simulink model "Sfunction_test"  (Simulink 8.5)
settings: Solver=ode45  StartTime=0.0  StopTime=7  RelTol=1e-3
undefined symbols (not defined in the file or in its folder): sample_time
settings Model: Creator=User  LastModifiedBy=User
settings DataIOCC: SignalLoggingSaveFormat=Dataset
settings OptimizationCC: ExpressionDepthLimit=128
settings DebuggingCC: UnderspecifiedInitializationDetection=Simplified  MergeDetectMultiDrivingBlocksExec=error  FcnCallInpInsideContextMsg=EnableAllAsError  StateNameClashWarn=none
settings GRTTargetCC: CombineOutputUpdateFcns=on  GRTInterface=off

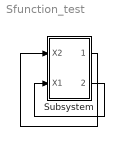
== system Sfunction_test ==
  Subsystem : Subsystem
  wires:
  Subsystem/2(x_1) -> Subsystem/2(X1)
  Subsystem/1(x_22) -> Subsystem/1(X2)

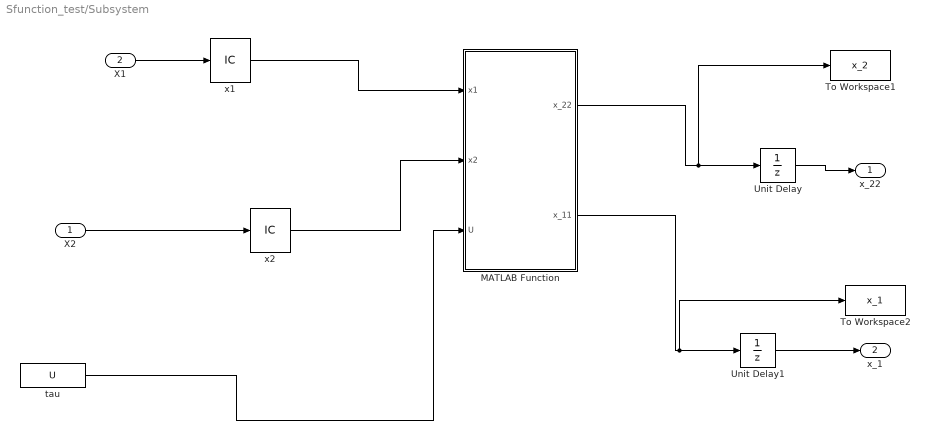
== system Sfunction_test/Subsystem ==
  X2 : Inport  PortDimensions=[7]
  X1 : Inport  Port=2  PortDimensions=[7]
  MATLAB Function : MATLAB Function  TreatAsAtomicUnit=on
  To Workspace1 : ToWorkspace  VariableName=x_2  SaveFormat=Structure With Time  SampleTime=-1
  To Workspace2 : ToWorkspace  VariableName=x_1  SaveFormat=Structure With Time  SampleTime=-1
  Unit Delay : UnitDelay  SampleTime=sample_time
  Unit Delay1 : UnitDelay  SampleTime=sample_time
  "tau " : FromWorkspace  VariableName=U  SampleTime=sample_time
  x1 : InitialCondition  Value=[-0.1106,-1.9490,-0.192,3.18400,0.2825,0.0969,-0.2798]
  x2 : InitialCondition  Value=[0 0 0 0 0 0 0]
  x_22 : Outport  PortDimensions=7
  x_1 : Outport  Port=2  PortDimensions=7
  wires:
  MATLAB Function/1(x_22) -> To Workspace1/1, Unit Delay/1
  MATLAB Function/2(x_11) -> To Workspace2/1, Unit Delay1/1
  "tau "/1 -> MATLAB Function/3(U)
  x1/1 -> MATLAB Function/1(x1)
  x2/1 -> MATLAB Function/2(x2)
  X2/1 -> x2/1
  X1/1 -> x1/1
  Unit Delay/1 -> x_22/1
  Unit Delay1/1 -> x_1/1

== matlab function Subsystem/MATLAB Function ==
  data: x1 input double; x_22 output double; x2 input double; U input double; x_11 output double
%
% gravComp7DOFNum Compute inverse dynamics via recursive Newton-Euler formulation
%
% Recursive Newton-Euler for standard Denavit-Hartenberg notation.
%

% Copyright (C) 1993-2011, by Peter I. Corke
%
% This file originally was part of The Robotics Toolbox for Matlab (RTB).
%
% http://www.petercorke.com

%
% Simplified from rne_dh for 7DOF WAM to compute only torque from gravity by Hans Vorsteveld
% Does not use structures from RTB, only the RNE algorithm
%

function [x_22,x_11] = PID(x1,x2,U)

%-------------------------------------------------------------------------------------
%   SETUP THE ARM
%-------------------------------------------------------------------------------------    
  Ts=0.002;
    



 
 
yd = [posd;veld];


        
         
         
        % In experimental work you do not add noise instead you only use measurement of position
        x_11 =  x2*Ts + x1; % Here we are estimating position using the extimate of x2 and measurement of x1 at present time
        
        %XX2 = (x_11-x_1)/Ts; 
        %XX2 = (x1-x1d)/Ts; 
        
        %x_22= (-inv(D(pos_meas))*((G(pos_meas)))+ inv(D(pos_meas))*U)*Ts + XX2 ;
        x3=(-inv(D(x1))*((G(x1)))+ inv(D(x1))*U);
       x_22=  x2 + Ts*x3;
        
        
        
    
   
end 

function G=G(q)


DH_a = [0 0 0.045 -0.045 0 0 0];
    DH_d = [0 0 .55 0 0.45 0 0.061];
    DH_alpha = [-pi/2 pi/2 -pi/2 pi/2 -pi/2 pi/2 0];

    m = [10.7676 3.87 1.8022 2.4 0.1237 0.4979886 0.07548270];
    
     
    com= zeros(3,7);
    
   com(:,1) = [-0.00443422;0.12189039;-0.00066489];
    com(:,2) = [-0.00236983;0.03105614;0.01542114 ];
    com(:,3) = [-0.03825858;0.20750770;0.00003309];
    com(:,4) = [0.00498512;-0.00022942;0.13271662 ];
    com(:,5) = [0.00008921;0.00511217;0.00435824];
    com(:,6) = [-0.00012262;-0.01703194;0.02468336];
    com(:,7) = [-0.00007974;0.00016313;-0.00323552 ];
     
     % hand_mass =1.385;
      %  DH_d(7) =DH_d(7)+ .0953; % Adding the distance to the hand frame for the Schunk Gripper
       % com(:,7) =(com(:,7).*hand_mass+com(:,7).*m(7))/(hand_mass+m(7)); % Finding the combined center of mass
        %m(7) =m(7)+hand_mass;  
        
    I=zeros(3,3,7);
    T=zeros(4,4,7);
     I(:,:,1) = [0.29486350,-0.00795023,-0.00009311;
                 -0.00795023,0.11350017,-0.00018711;
                -0.00009311,-0.00018711,0.25065343];
    I(:,:,2) =[0.02606840,-0.00001346,-0.00011701;
               -0.00001346,0.01472202,0.00003659;
              -0.00011701,0.00003659,0.01934814];
    I(:,:,3) = [0.13671601,-0.01680434, 0.00000510;
               -0.01680434,0.00588354,-0.00000530;
                0.00000510,-0.00000530,0.13951371];
    I(:,:,4) = [ 0.05719268,0.00001467,0.00008193;
                 0.00001467,0.05716470,-0.00009417;
                 0.00008193,-0.00009417,0.00300441] ;
    I(:,:,5) =[0.00005587,0.00000026,.00000000;
               0.00000026,0.00007817,-0.00000083;
               0.00000000,-0.00000083,0.00006594];
    I(:,:,6) = [0.00093106,0.00000148,-0.00000201;
                0.00000148, 0.00049833,-0.00022162;
               -0.00000201,-0.00022162,0.00057483];
    I(:,:,7) = [0.003167342, 0,0;       % Approximate Inertia Tensor for Schunk Gripper
                0,0.001128942,0;
                 0,0,0.00258007;];  
            
             
for j=1:7,
        a = DH_a(j);
        d = DH_d(j);
        alpha = DH_alpha(j);
        T(:,:,j) = getTransformDH(a, d, alpha, q(j));
end 


comstar=zeros(4,7);

   
    comstar(:,1) = [com(:,1);1];
    comstar(:,2) = [com(:,2);1];
    comstar(:,3) = [com(:,3);1];
    comstar(:,4) = [com(:,4);1];
    comstar(:,5) = [com(:,5);1];
    comstar(:,6) = [com(:,6);1];
    comstar(:,7) = [com(:,7);1];
    
    Q=zeros(4,4);
    
    Q=[0,-1,0,0;
     1,0,0,0;
     0,0,0,0;
     0,0,0,0];
   
 gravity=[0,0,-9.81,0];
 G=zeros(7,1)
 
   G(1)= -m(1)*gravity*Q*T(:,:,1)*comstar(:,1)-m(2)*gravity*Q*T(:,:,1)*T(:,:,2)*comstar(:,2)-m(3)*gravity*Q*T(:,:,1)*T(:,:,2)*T(:,:,3)*comstar(:,3)-m(4)*gravity*Q*T(:,:,1)*T(:,:,2)*T(:,:,3)*T(:,:,4)*comstar(:,4)-m(5)*gravity*Q*T(:,:,1)*T(:,:,2)*T(:,:,3)*T(:,:,4)*T(:,:,5)*comstar(:,5)-m(6)*gravity*Q*T(:,:,1)*T(:,:,2)*T(:,:,3)*T(:,:,4)*T(:,:,5)*T(:,:,6)*comstar(:,6)-m(7)*gravity*Q*T(:,:,1)*T(:,:,2)*T(:,:,3)*T(:,:,4)*T(:,:,5)*T(:,:,6)*T(:,:,7)*comstar(:,7);   
   G(2)= -m(2)*gravity*T(:,:,1)*Q*T(:,:,2)*comstar(:,2)-m(3)*gravity*T(:,:,1)*Q*T(:,:,2)*T(:,:,3)*comstar(:,3)-m(4)*gravity*T(:,:,1)*Q*T(:,:,2)*T(:,:,3)*T(:,:,4)*comstar(:,4)-m(5)*gravity*T(:,:,1)*Q*T(:,:,2)*T(:,:,3)*T(:,:,4)*T(:,:,5)*comstar(:,5)-m(6)*gravity*T(:,:,1)*Q*T(:,:,2)*T(:,:,3)*T(:,:,4)*T(:,:,5)*T(:,:,6)*comstar(:,6)-m(7)*gravity*T(:,:,1)*Q*T(:,:,2)*T(:,:,3)*T(:,:,4)*T(:,:,5)*T(:,:,6)*T(:,:,7)*comstar(:,7);
   G(3)= -m(3)*gravity*T(:,:,1)*T(:,:,2)*Q*T(:,:,3)*comstar(:,3)-m(4)*gravity*T(:,:,1)*T(:,:,2)*Q*T(:,:,3)*T(:,:,4)*comstar(:,4)-m(5)*gravity*T(:,:,1)*T(:,:,2)*Q*T(:,:,3)*T(:,:,4)*T(:,:,5)*comstar(:,5)-m(6)*gravity*T(:,:,1)*T(:,:,2)*Q*T(:,:,3)*T(:,:,4)*T(:,:,5)*T(:,:,6)*comstar(:,6)-m(7)*gravity*T(:,:,1)*T(:,:,2)*Q*T(:,:,3)*T(:,:,4)*T(:,:,5)*T(:,:,6)*T(:,:,7)*comstar(:,7);
   G(4)= -m(4)*gravity*T(:,:,1)*T(:,:,2)*T(:,:,3)*Q*T(:,:,4)*comstar(:,4)-m(5)*gravity*T(:,:,1)*T(:,:,2)*T(:,:,3)*Q*T(:,:,4)*T(:,:,5)*comstar(:,5)-m(6)*gravity*T(:,:,1)*T(:,:,2)*T(:,:,3)*Q*T(:,:,4)*T(:,:,5)*T(:,:,6)*comstar(:,6)-m(7)*gravity*T(:,:,1)*T(:,:,2)*T(:,:,3)*Q*T(:,:,4)*T(:,:,5)*T(:,:,6)*T(:,:,7)*comstar(:,7);
   G(5)= -m(5)*gravity*T(:,:,1)*T(:,:,2)*T(:,:,3)*T(:,:,4)*Q*T(:,:,5)*comstar(:,5)-m(6)*gravity*T(:,:,1)*T(:,:,2)*T(:,:,3)*T(:,:,4)*Q*T(:,:,5)*T(:,:,6)*comstar(:,6)-m(7)*gravity*T(:,:,1)*T(:,:,2)*T(:,:,3)*T(:,:,4)*Q*T(:,:,5)*T(:,:,6)*T(:,:,7)*comstar(:,7);
   G(6)= -m(6)*gravity*T(:,:,1)*T(:,:,2)*T(:,:,3)*T(:,:,4)*T(:,:,5)*Q*T(:,:,6)*comstar(:,6)-m(7)*gravity*T(:,:,1)*T(:,:,2)*T(:,:,3)*T(:,:,4)*T(:,:,5)*Q*T(:,:,6)*T(:,:,7)*comstar(:,7);
   G(7)= -m(7)*gravity*T(:,:,1)*T(:,:,2)*T(:,:,3)*T(:,:,4)*T(:,:,5)*T(:,:,6)*Q*T(:,:,7)*comstar(:,7);
    
end 

function D =D(q);
DH_a = [0 0 0.045 -0.045 0 0 0];
    DH_d = [0 0 .55 0 0.45 0 0.061];
    DH_alpha = [-pi/2 pi/2 -pi/2 pi/2 -pi/2 pi/2 0];

    m = [10.7676 3.87 1.8022 2.4 0.1237 0.4979886 0.07548270];
    
     
    com= zeros(3,7);
    
   com(:,1) = [-0.00443422;0.12189039;-0.00066489];
    com(:,2) = [-0.00236983;0.03105614;0.01542114 ];
    com(:,3) = [-0.03825858;0.20750770;0.00003309];
    com(:,4) = [0.00498512;-0.00022942;0.13271662 ];
    com(:,5) = [0.00008921;0.00511217;0.00435824];
    com(:,6) = [-0.00012262;-0.01703194;0.02468336];
    com(:,7) = [-0.00007974;0.00016313;-0.00323552 ];
     
       
        
    I=zeros(3,3,7);
    T=zeros(4,4,7);
     I(:,:,1) = [0.29486350,-0.00795023,-0.00009311;
                 -0.00795023,0.11350017,-0.00018711;
                -0.00009311,-0.00018711,0.25065343];
    I(:,:,2) =[0.02606840,-0.00001346,-0.00011701;
               -0.00001346,0.01472202,0.00003659;
              -0.00011701,0.00003659,0.01934814];
    I(:,:,3) = [0.13671601,-0.01680434, 0.00000510;
               -0.01680434,0.00588354,-0.00000530;
                0.00000510,-0.00000530,0.13951371];
    I(:,:,4) = [ 0.05719268,0.00001467,0.00008193;
                 0.00001467,0.05716470,-0.00009417;
                 0.00008193,-0.00009417,0.00300441] ;
    I(:,:,5) =[0.00005587,0.00000026,.00000000;
               0.00000026,0.00007817,-0.00000083;
               0.00000000,-0.00000083,0.00006594];
    I(:,:,6) = [0.00093106,0.00000148,-0.00000201;
                0.00000148, 0.00049833,-0.00022162;
               -0.00000201,-0.00022162,0.00057483];
    I(:,:,7) = [0.003167342, 0,0;       % Approximate Inertia Tensor for Schunk Gripper
                0,0.001128942,0;
                 0,0,0.00258007;];  
            
             
             
for j=1:7,
        a = DH_a(j);
        d = DH_d(j);
        alpha = DH_alpha(j);
        T(:,:,j) = getTransformDH(a, d, alpha, q(j));
end 

comstar=zeros(4,7);

   
    comstar(:,1) = [com(:,1);1];
    comstar(:,2) = [com(:,2);1];
    comstar(:,3) = [com(:,3);1];
    comstar(:,4) = [com(:,4);1];
    comstar(:,5) = [com(:,5);1];
    comstar(:,6) = [com(:,6);1];
    comstar(:,7) = [com(:,7);1];
    
    Q=zeros(4,4);
    
    Q=[0,-1,0,0;
     1,0,0,0;
     0,0,0,0;
     0,0,0,0];
   

   
U=zeros(4,4,7,7);
   
   U(:,:,1,1)= Q*T(:,:,1);
   U(:,:,2,1)= Q*T(:,:,1)*T(:,:,2);
   U(:,:,3,1)= Q*T(:,:,1)*T(:,:,2)*T(:,:,3);
   U(:,:,4,1)= Q*T(:,:,1)*T(:,:,2)*T(:,:,3)*T(:,:,4);
   U(:,:,5,1)= Q*T(:,:,1)*T(:,:,2)*T(:,:,3)*T(:,:,4)*T(:,:,5);
   U(:,:,6,1)= Q*T(:,:,1)*T(:,:,2)*T(:,:,3)*T(:,:,4)*T(:,:,5)*T(:,:,6);
   U(:,:,7,1)= Q*T(:,:,1)*T(:,:,2)*T(:,:,3)*T(:,:,4)*T(:,:,5)*T(:,:,6)*T(:,:,7);
   
   
   U(:,:,2,2)= T(:,:,1)*Q*T(:,:,2);
   U(:,:,3,2)= T(:,:,1)*Q*T(:,:,2)*T(:,:,3);
   U(:,:,4,2)= T(:,:,1)*Q*T(:,:,2)*T(:,:,3)*T(:,:,4);
   U(:,:,5,2)= T(:,:,1)*Q*T(:,:,2)*T(:,:,3)*T(:,:,4)*T(:,:,5);
   U(:,:,6,2)= T(:,:,1)*Q*T(:,:,2)*T(:,:,3)*T(:,:,4)*T(:,:,5)*T(:,:,6);
   U(:,:,7,2)= T(:,:,1)*Q*T(:,:,2)*T(:,:,3)*T(:,:,4)*T(:,:,5)*T(:,:,6)*T(:,:,7);
   
  
   U(:,:,3,3)= T(:,:,1)*T(:,:,2)*Q*T(:,:,3);
   U(:,:,4,3)= T(:,:,1)*T(:,:,2)*Q*T(:,:,3)*T(:,:,4);
   U(:,:,5,3)= T(:,:,1)*T(:,:,2)*Q*T(:,:,3)*T(:,:,4)*T(:,:,5);
   U(:,:,6,3)= T(:,:,1)*T(:,:,2)*Q*T(:,:,3)*T(:,:,4)*T(:,:,5)*T(:,:,6);
   U(:,:,7,3)= T(:,:,1)*T(:,:,2)*Q*T(:,:,3)*T(:,:,4)*T(:,:,5)*T(:,:,6)*T(:,:,7);
   
   U(:,:,4,4)= T(:,:,1)*T(:,:,2)*T(:,:,3)*Q*T(:,:,4);
   U(:,:,5,4)= T(:,:,1)*T(:,:,2)*T(:,:,3)*Q*T(:,:,4)*T(:,:,5);
   U(:,:,6,4)= T(:,:,1)*T(:,:,2)*T(:,:,3)*Q*T(:,:,4)*T(:,:,5)*T(:,:,6);
   U(:,:,7,4)= T(:,:,1)*T(:,:,2)*T(:,:,3)*Q*T(:,:,4)*T(:,:,5)*T(:,:,6)*T(:,:,7);
   
   U(:,:,5,5)= T(:,:,1)*T(:,:,2)*T(:,:,3)*T(:,:,4)*Q*T(:,:,5);
   U(:,:,6,5)= T(:,:,1)*T(:,:,2)*T(:,:,3)*T(:,:,4)*Q*T(:,:,5)*T(:,:,6);
   U(:,:,7,5)= T(:,:,1)*T(:,:,2)*T(:,:,3)*T(:,:,4)*Q*T(:,:,5)*T(:,:,6)*T(:,:,7);
   
   U(:,:,6,6)= T(:,:,1)*T(:,:,2)*T(:,:,3)*T(:,:,4)*T(:,:,5)*Q*T(:,:,6);
   U(:,:,7,6)= T(:,:,1)*T(:,:,2)*T(:,:,3)*T(:,:,4)*T(:,:,5)*Q*T(:,:,6)*T(:,:,7);
   
   U(:,:,7,7)= T(:,:,1)*T(:,:,2)*T(:,:,3)*T(:,:,4)*T(:,:,5)*T(:,:,6)*Q*T(:,:,7);
   
   
   
  
   J=zeros(4,4,7);
 
   
   J(:,:,1)=[0.5*(-I(1,1,1)+I(2,2,1)+I(3,3,1)), I(1,2,1), I(1,3,1), m(1)*com(1,1);
             I(1,2,1) ,0.5*(I(1,1,1)-I(2,2,1)+I(3,3,1)), I(2,3,1), m(1)*com(2,1);
             I(1,3,1), I(2,3,1), 0.5*(I(1,1,1)+I(2,2,1)-I(3,3,1)), m(1)*com(3,1);
              m(1)*com(1,1), m(1)*com(2,1), m(1)*com(3,1), m(1)];
   
    J(:,:,2)=[0.5*(-I(1,1,2)+I(2,2,2)+I(3,3,2)), I(1,2,2), I(1,3,2), m(2)*com(1,2);
             I(1,2,2) ,0.5*(I(1,1,2)-I(2,2,2)+I(3,3,2)), I(2,3,2), m(2)*com(2,2);
             I(1,3,2), I(2,3,2), 0.5*(I(1,1,2)+I(2,2,2)-I(3,3,2)), m(2)*com(3,2);
              m(2)*com(1,2), m(2)*com(2,2), m(2)*com(3,2), m(2)];
   
          
     J(:,:,3)=[0.5*(-I(1,1,3)+I(2,2,3)+I(3,3,3)), I(1,2,3), I(1,3,3), m(3)*com(1,3);
             I(1,2,3) ,0.5*(I(1,1,3)-I(2,2,3)+I(3,3,3)), I(2,3,3), m(3)*com(2,3);
             I(1,3,3), I(2,3,3), 0.5*(I(1,1,3)+I(2,2,3)-I(3,3,3)), m(3)*com(3,3);
              m(3)*com(1,3), m(3)*com(2,3), m(3)*com(3,3), m(3)];      
   
   
    J(:,:,4)=[0.5*(-I(1,1,4)+I(2,2,4)+I(3,3,4)), I(1,2,4), I(1,3,4), m(4)*com(1,4);
             I(1,2,4) ,0.5*(I(1,1,4)-I(2,2,4)+I(3,3,4)), I(2,3,4), m(4)*com(2,4);
             I(1,3,4), I(2,3,4), 0.5*(I(1,1,4)+I(2,2,4)-I(3,3,4)), m(4)*com(3,4);
              m(4)*com(1,4), m(4)*com(2,4), m(4)*com(3,4), m(4)];
   
   
    J(:,:,5)=[0.5*(-I(1,1,5)+I(2,2,5)+I(3,3,5)), I(1,2,5), I(1,3,5), m(5)*com(1,5);
             I(1,2,5) ,0.5*(I(1,1,5)-I(2,2,5)+I(3,3,5)), I(2,3,5), m(5)*com(2,5);
             I(1,3,5), I(2,3,5), 0.5*(I(1,1,5)+I(2,2,5)-I(3,3,5)), m(5)*com(3,5);
              m(5)*com(1,5), m(5)*com(2,5), m(5)*com(3,5), m(5)];
   
   
    J(:,:,6)=[0.5*(-I(1,1,6)+I(2,2,6)+I(3,3,6)), I(1,2,6), I(1,3,6), m(6)*com(1,6);
             I(1,2,6) ,0.5*(I(1,1,6)-I(2,2,6)+I(3,3,6)), I(2,3,6), m(6)*com(2,6);
             I(1,3,6), I(2,3,6), 0.5*(I(1,1,6)+I(2,2,6)-I(3,3,6)), m(6)*com(3,6);
              m(6)*com(1,6), m(6)*com(2,6), m(6)*com(3,6), m(6)];
   
   
    J(:,:,7)=[0.5*(-I(1,1,7)+I(2,2,7)+I(3,3,7)), I(1,2,7), I(1,3,7), m(7)*com(1,7);
             I(1,2,7) ,0.5*(I(1,1,7)-I(2,2,7)+I(3,3,7)), I(2,3,7), m(7)*com(2,7);
             I(1,3,7), I(2,3,7), 0.5*(I(1,1,7)+I(2,2,7)-I(3,3,7)), m(7)*com(3,7);
              m(7)*com(1,7), m(7)*com(2,7), m(7)*com(3,7), m(7)];
          
          D=zeros(7,7);
   
   
    D(1,1)= trace(U(:,:,1,1)*J(:,:,1)*transpose(U(:,:,1,1))) + trace(U(:,:,2,1)*J(:,:,2)*transpose(U(:,:,2,1))) + trace(U(:,:,3,1)*J(:,:,3)*transpose(U(:,:,3,1))) + trace(U(:,:,4,1)*J(:,:,4)*transpose(U(:,:,4,1))) + trace(U(:,:,5,1)*J(:,:,5)*transpose(U(:,:,5,1))) + trace(U(:,:,6,1)*J(:,:,6)*transpose(U(:,:,6,1))) + trace(U(:,:,7,1)*J(:,:,7)*transpose(U(:,:,7,1))) ;
    D(1,2)= trace(U(:,:,2,2)*J(:,:,2)*transpose(U(:,:,2,1))) + trace(U(:,:,3,2)*J(:,:,3)*transpose(U(:,:,3,1))) + trace(U(:,:,4,2)*J(:,:,4)*transpose(U(:,:,4,1))) +trace(U(:,:,5,2)*J(:,:,5)*transpose(U(:,:,5,1))) + trace(U(:,:,6,2)*J(:,:,6)*transpose(U(:,:,6,1))) + trace(U(:,:,7,2)*J(:,:,7)*transpose(U(:,:,7,1))); 
    D(1,3)= trace(U(:,:,3,3)*J(:,:,3)*transpose(U(:,:,3,1)))+ trace(U(:,:,4,3)*J(:,:,4)*transpose(U(:,:,4,1)))+ trace(U(:,:,5,3)*J(:,:,5)*transpose(U(:,:,5,1)))+ trace(U(:,:,6,3)*J(:,:,6)*transpose(U(:,:,6,1)))+ trace(U(:,:,7,3)*J(:,:,7)*transpose(U(:,:,7,1))); 
    D(1,4)= trace(U(:,:,4,4)*J(:,:,4)*transpose(U(:,:,4,1)))+ trace(U(:,:,5,4)*J(:,:,5)*transpose(U(:,:,5,1)))+ trace(U(:,:,6,4)*J(:,:,6)*transpose(U(:,:,6,1)))+ trace(U(:,:,7,4)*J(:,:,7)*transpose(U(:,:,7,1)));
    D(1,5)= trace(U(:,:,5,5)*J(:,:,5)*transpose(U(:,:,5,1)))+ trace(U(:,:,6,5)*J(:,:,6)*transpose(U(:,:,6,1)))+ trace(U(:,:,7,5)*J(:,:,7)*transpose(U(:,:,7,1)));
    D(1,6)= trace(U(:,:,6,6)*J(:,:,6)*transpose(U(:,:,6,1)))+ trace(U(:,:,7,6)*J(:,:,7)*transpose(U(:,:,7,1)));
    D(1,7)= trace(U(:,:,7,7)*J(:,:,7)*transpose(U(:,:,7,1)));
    
    D(2,1)= trace(U(:,:,2,1)*J(:,:,2)*transpose(U(:,:,2,2)))+ trace(U(:,:,3,1)*J(:,:,3)*transpose(U(:,:,3,2)))+ trace(U(:,:,4,1)*J(:,:,4)*transpose(U(:,:,4,2)))+ trace(U(:,:,5,1)*J(:,:,5)*transpose(U(:,:,5,2)))+ trace(U(:,:,6,1)*J(:,:,6)*transpose(U(:,:,6,2)))+ trace(U(:,:,7,1)*J(:,:,7)*transpose(U(:,:,7,2)));
    D(2,2)= trace(U(:,:,2,2)*J(:,:,2)*transpose(U(:,:,2,2)))+ trace(U(:,:,3,2)*J(:,:,3)*transpose(U(:,:,3,2)))+ trace(U(:,:,4,2)*J(:,:,4)*transpose(U(:,:,4,2)))+ trace(U(:,:,5,2)*J(:,:,5)*transpose(U(:,:,5,2)))+ trace(U(:,:,6,2)*J(:,:,6)*transpose(U(:,:,6,2)))+ trace(U(:,:,7,2)*J(:,:,7)*transpose(U(:,:,7,2)));
    D(2,3)= trace(U(:,:,3,3)*J(:,:,3)*transpose(U(:,:,3,2)))+ trace(U(:,:,4,3)*J(:,:,4)*transpose(U(:,:,4,2)))+ trace(U(:,:,5,3)*J(:,:,5)*transpose(U(:,:,5,2)))+ trace(U(:,:,6,3)*J(:,:,6)*transpose(U(:,:,6,2)))+ trace(U(:,:,7,3)*J(:,:,7)*transpose(U(:,:,7,2))); 
    D(2,4)= trace(U(:,:,4,4)*J(:,:,4)*transpose(U(:,:,4,2)))+ trace(U(:,:,5,4)*J(:,:,5)*transpose(U(:,:,5,2)))+ trace(U(:,:,6,4)*J(:,:,6)*transpose(U(:,:,6,2)))+ trace(U(:,:,7,4)*J(:,:,7)*transpose(U(:,:,7,2))); 
    D(2,5)= trace(U(:,:,5,5)*J(:,:,5)*transpose(U(:,:,5,2)))+ trace(U(:,:,6,5)*J(:,:,6)*transpose(U(:,:,6,2)))+ trace(U(:,:,7,5)*J(:,:,7)*transpose(U(:,:,7,2)));
    D(2,6)= trace(U(:,:,6,6)*J(:,:,6)*transpose(U(:,:,6,2)))+ trace(U(:,:,7,6)*J(:,:,7)*transpose(U(:,:,7,2))); 
    D(2,7)= trace(U(:,:,7,7)*J(:,:,7)*transpose(U(:,:,7,2)));
  
    D(3,1)= trace(U(:,:,3,1)*J(:,:,3)*transpose(U(:,:,3,3)))+ trace(U(:,:,4,1)*J(:,:,4)*transpose(U(:,:,4,3)))+ trace(U(:,:,5,1)*J(:,:,5)*transpose(U(:,:,5,3)))+ trace(U(:,:,6,1)*J(:,:,6)*transpose(U(:,:,6,3)))+ trace(U(:,:,7,1)*J(:,:,7)*transpose(U(:,:,7,3)));
    D(3,2)= trace(U(:,:,3,2)*J(:,:,3)*transpose(U(:,:,3,3)))+ trace(U(:,:,4,2)*J(:,:,4)*transpose(U(:,:,4,3)))+ trace(U(:,:,5,2)*J(:,:,5)*transpose(U(:,:,5,3)))+ trace(U(:,:,6,2)*J(:,:,6)*transpose(U(:,:,6,3)))+ trace(U(:,:,7,2)*J(:,:,7)*transpose(U(:,:,7,3)));
    D(3,3)= trace(U(:,:,3,3)*J(:,:,3)*transpose(U(:,:,3,3)))+ trace(U(:,:,4,3)*J(:,:,4)*transpose(U(:,:,4,3)))+ trace(U(:,:,5,3)*J(:,:,5)*transpose(U(:,:,5,3)))+ trace(U(:,:,6,3)*J(:,:,6)*transpose(U(:,:,6,3)))+ trace(U(:,:,7,3)*J(:,:,7)*transpose(U(:,:,7,3)));
    D(3,4)= trace(U(:,:,4,4)*J(:,:,4)*transpose(U(:,:,4,3)))+ trace(U(:,:,5,4)*J(:,:,5)*transpose(U(:,:,5,3)))+ trace(U(:,:,6,4)*J(:,:,6)*transpose(U(:,:,6,3)))+ trace(U(:,:,7,4)*J(:,:,7)*transpose(U(:,:,7,3)));
    D(3,5)= trace(U(:,:,5,5)*J(:,:,5)*transpose(U(:,:,5,3)))+ trace(U(:,:,6,5)*J(:,:,6)*transpose(U(:,:,6,3)))+ trace(U(:,:,7,5)*J(:,:,7)*transpose(U(:,:,7,3)));
    D(3,6)= trace(U(:,:,6,6)*J(:,:,6)*transpose(U(:,:,6,3)))+ trace(U(:,:,7,6)*J(:,:,7)*transpose(U(:,:,7,3)));
    D(3,7)= trace(U(:,:,7,7)*J(:,:,7)*transpose(U(:,:,7,3)));
     
     
    D(4,1)= trace(U(:,:,4,1)*J(:,:,4)*transpose(U(:,:,4,4)))+ trace(U(:,:,5,1)*J(:,:,5)*transpose(U(:,:,5,4)))+ trace(U(:,:,6,1)*J(:,:,6)*transpose(U(:,:,6,4)))+ trace(U(:,:,7,1)*J(:,:,7)*transpose(U(:,:,7,4))); 
    D(4,2)= trace(U(:,:,4,2)*J(:,:,4)*transpose(U(:,:,4,4)))+ trace(U(:,:,5,2)*J(:,:,5)*transpose(U(:,:,5,4)))+ trace(U(:,:,6,2)*J(:,:,6)*transpose(U(:,:,6,4)))+ trace(U(:,:,7,2)*J(:,:,7)*transpose(U(:,:,7,4))); 
    D(4,3)= trace(U(:,:,4,3)*J(:,:,4)*transpose(U(:,:,4,4)))+ trace(U(:,:,5,3)*J(:,:,5)*transpose(U(:,:,5,4)))+ trace(U(:,:,6,3)*J(:,:,6)*transpose(U(:,:,6,4)))+ trace(U(:,:,7,3)*J(:,:,7)*transpose(U(:,:,7,4)));
    D(4,4)= trace(U(:,:,4,4)*J(:,:,4)*transpose(U(:,:,4,4)))+ trace(U(:,:,5,4)*J(:,:,5)*transpose(U(:,:,5,4)))+ trace(U(:,:,6,4)*J(:,:,6)*transpose(U(:,:,6,4)))+ trace(U(:,:,7,4)*J(:,:,7)*transpose(U(:,:,7,4)));
    D(4,5)= trace(U(:,:,5,5)*J(:,:,5)*transpose(U(:,:,5,4)))+ trace(U(:,:,6,5)*J(:,:,6)*transpose(U(:,:,6,4)))+ trace(U(:,:,7,5)*J(:,:,7)*transpose(U(:,:,7,4)));
    D(4,6)= trace(U(:,:,6,6)*J(:,:,6)*transpose(U(:,:,6,4)))+ trace(U(:,:,7,6)*J(:,:,7)*transpose(U(:,:,7,4))); 
    D(4,7)= trace(U(:,:,7,7)*J(:,:,7)*transpose(U(:,:,7,4)));
    
    D(5,1)= trace(U(:,:,5,1)*J(:,:,5)*transpose(U(:,:,5,5)))+ trace(U(:,:,6,1)*J(:,:,6)*transpose(U(:,:,6,5)))+ trace(U(:,:,7,1)*J(:,:,7)*transpose(U(:,:,7,5)));
    D(5,2)= trace(U(:,:,5,2)*J(:,:,5)*transpose(U(:,:,5,5)))+ trace(U(:,:,6,2)*J(:,:,6)*transpose(U(:,:,6,5)))+ trace(U(:,:,7,2)*J(:,:,7)*transpose(U(:,:,7,5)));
    D(5,3)= trace(U(:,:,5,3)*J(:,:,5)*transpose(U(:,:,5,5)))+ trace(U(:,:,6,3)*J(:,:,6)*transpose(U(:,:,6,5)))+ trace(U(:,:,7,3)*J(:,:,7)*transpose(U(:,:,7,5))); 
    D(5,4)= trace(U(:,:,5,4)*J(:,:,5)*transpose(U(:,:,5,5)))+ trace(U(:,:,6,4)*J(:,:,6)*transpose(U(:,:,6,5)))+ trace(U(:,:,7,4)*J(:,:,7)*transpose(U(:,:,7,5))); 
    D(5,5)= trace(U(:,:,5,5)*J(:,:,5)*transpose(U(:,:,5,5)))+ trace(U(:,:,6,5)*J(:,:,6)*transpose(U(:,:,6,5)))+ trace(U(:,:,7,5)*J(:,:,7)*transpose(U(:,:,7,5)));
    D(5,6)= trace(U(:,:,6,6)*J(:,:,6)*transpose(U(:,:,6,5)))+ trace(U(:,:,7,6)*J(:,:,7)*transpose(U(:,:,7,5))); 
    D(5,7)= trace(U(:,:,7,7)*J(:,:,7)*transpose(U(:,:,7,5)));
    
    D(6,1)= trace(U(:,:,6,1)*J(:,:,6)*transpose(U(:,:,6,6)))+ trace(U(:,:,7,1)*J(:,:,7)*transpose(U(:,:,7,6)));
    D(6,2)= trace(U(:,:,6,2)*J(:,:,6)*transpose(U(:,:,6,6)))+ trace(U(:,:,7,2)*J(:,:,7)*transpose(U(:,:,7,6)));
    D(6,3)= trace(U(:,:,6,3)*J(:,:,6)*transpose(U(:,:,6,6)))+ trace(U(:,:,7,3)*J(:,:,7)*transpose(U(:,:,7,6))); 
    D(6,4)= trace(U(:,:,6,4)*J(:,:,6)*transpose(U(:,:,6,6)))+ trace(U(:,:,7,4)*J(:,:,7)*transpose(U(:,:,7,6))); 
    D(6,5)= trace(U(:,:,6,5)*J(:,:,6)*transpose(U(:,:,6,6)))+ trace(U(:,:,7,5)*J(:,:,7)*transpose(U(:,:,7,6))); 
    D(6,6)= trace(U(:,:,6,6)*J(:,:,6)*transpose(U(:,:,6,6)))+ trace(U(:,:,7,6)*J(:,:,7)*transpose(U(:,:,7,6))); 
    D(6,7)= trace(U(:,:,7,7)*J(:,:,7)*transpose(U(:,:,7,6)));
    
    D(7,1)= trace(U(:,:,7,1)*J(:,:,7)*transpose(U(:,:,7,7)));
    D(7,2)= trace(U(:,:,7,2)*J(:,:,7)*transpose(U(:,:,7,7)));
    D(7,3)= trace(U(:,:,7,3)*J(:,:,7)*transpose(U(:,:,7,7)));
    D(7,4)= trace(U(:,:,7,4)*J(:,:,7)*transpose(U(:,:,7,7)));
    D(7,5)= trace(U(:,:,7,5)*J(:,:,7)*transpose(U(:,:,7,7)));
    D(7,6)= trace(U(:,:,7,6)*J(:,:,7)*transpose(U(:,:,7,7)));
    D(7,7)= trace(U(:,:,7,7)*J(:,:,7)*transpose(U(:,:,7,7)));
end 


 function T = getTransformDH(a,d,alpha,q)
    ct = cos(q);
    st = sin(q);
    cb = cos(alpha);
    sb = sin(alpha);
    
    T = [ ct, -st*cb,  st*sb, a*ct;
          st,  ct*cb, -ct*sb, a*st;
          0, sb, cb, d;
          0, 0, 0, 1 ];            
 end
